simulink model "Traking_step"  (R2019a)
settings: Solver=VariableStepAuto  StartTime=0.0  StopTime=10.0  RelTol=1e-3
values from neighbouring files (symbols this model uses):
  den = Gcl.Denominator{1, 1}    [Step_plot.m]
  num = Gcl.Numerator{1, 1}    [Step_plot.m]
settings Model: Creator=xde12  LastModifiedBy=xde12

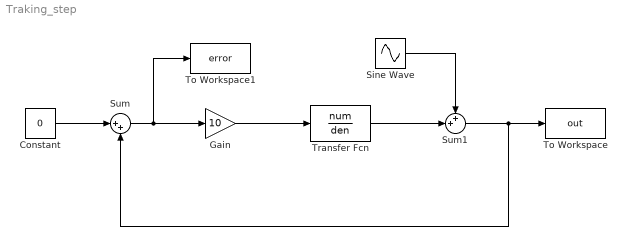
== system Traking_step ==
  Constant : Constant  Value=0
  Gain : Gain  Gain=10
  Sine Wave : Sin  Amplitude=300  Frequency=0.5  SampleTime=0
  Sum : Sum  Inputs=|++
  Sum1 : Sum  Inputs=++|
  To Workspace : ToWorkspace  VariableName=out  SaveFormat=Structure With Time  SampleTime=-1
  To Workspace1 : ToWorkspace  VariableName=error  SaveFormat=Structure With Time  SampleTime=-1
  Transfer Fcn : TransferFcn  Numerator=num  Denominator=den
  wires:
  Gain/1 -> Transfer Fcn/1
  Constant/1 -> Sum/1
  Sum/1 -> To Workspace1/1, Gain/1
  Transfer Fcn/1 -> Sum1/2
  Sum1/1 -> Sum/2, To Workspace/1
  Sine Wave/1 -> Sum1/1
